simulink model "ExerciseModel_18072025"  (R2025a)
settings: Solver=ode4  StartTime=0.0  StopTime=tsim  FixedStep=1  RelTol=1e-3
model workspace (MAT data in the model file):
  step_size = 1
values from neighbouring files (symbols this model uses):
  A_w = [cosd(beta1)*sind(alfa1)  -cosd(beta2)*sind(alfa2) -cosd(beta3)*sind(alfa3) cosd(beta4)*sind(alfa4) ... (first row only)    [initfun_18072025.m]    (also in initfun_18072025_nogyro.m)
  A_wP = pinv(A_w)    [initfun_18072025.m]    (also in initfun_18072025_nogyro.m)
  ARW = deg2rad(0.23)/sqrt(3600)    [initfun_18072025.m]
  Bias = deg2rad(1)/3600    [initfun_18072025.m]
  C_d = 2.2    [initfun_18072025.m]    (also in initfun_18072025_nogyro.m)
  d_max = 0.29    [initfun_18072025.m]    (also in initfun_18072025_nogyro.m)
  d_min = 0    [initfun_18072025.m]    (also in initfun_18072025_nogyro.m)
  ET0 = cspice_str2et(Date_UTC)    [initfun_18072025.m]    (also in initfun_18072025_nogyro.m)
  FOV = 166    [initfun_18072025.m]    (also in initfun_18072025_nogyro.m)
  G_earth = 6.6742e-11    [initfun_18072025.m]    (also in initfun_18072025_nogyro.m)
  init_state = [initial_position,initial_velocity,ang_vel_init2,quat_0]'    [initfun_18072025.m]    (also in initfun_18072025_nogyro.m)
  K = [F Z(:); Z(:)' sigma]    [Gain_matrix.m]    (also in QUEST.m = Gain_matrix(V',W',a); initfun_18072025.m = schmidt(nmax, mmax); initfun_18072025_nogyro.m = schmidt(nmax, mmax))
  K_dp = K_d_pitch_1    [evaluate_gains.m]    (also in evaluate_gains_nogyro.m)
  K_dr = K_d_roll_1    [evaluate_gains.m]    (also in evaluate_gains_nogyro.m)
  K_dy = K_d_yaw_1    [evaluate_gains.m]    (also in evaluate_gains_nogyro.m)
  K_pp = K_p_pitch_1    [evaluate_gains.m]    (also in evaluate_gains_nogyro.m; initfun_18072025_nogyro.m = K_pp/2)
  K_pr = K_p_roll_1    [evaluate_gains.m]    (also in evaluate_gains_nogyro.m; initfun_18072025.m = K_pr*1.8)
  K_py = K_p_yaw_1    [evaluate_gains.m]    (also in evaluate_gains_nogyro.m; initfun_18072025.m = K_py*10)
  m_earth = 5.9736e24    (= 5.9736e+24)    [initfun_18072025.m]    (also in initfun_18072025_nogyro.m)
  Magnetic_dipole = [0.1; 0.1;  0.1]    [initfun_18072025.m]    (also in initfun_18072025_nogyro.m)
  Magnetometers_number = 2    [initfun_18072025.m]    (also in initfun_18072025_nogyro.m)
  Mean_cart_Mag = 0    [initfun_18072025.m]    (also in initfun_18072025_nogyro.m)
  MeanangularSun = 0    [initfun_18072025.m]    (also in initfun_18072025_nogyro.m)
  mmax = 3    [initfun_18072025.m]    (also in initfun_18072025_nogyro.m)
  nmax = 3    [initfun_18072025.m]    (also in initfun_18072025_nogyro.m)
  omegaOrb = [0;-2*pi/P;0]    [initfun_18072025.m]    (also in initfun_18072025_nogyro.m)
  P_prev = [P_dg, zeros(3,3) ... (first row only)    [initfun_18072025.m]    (also in initfun_18072025_nogyro.m)
  P_sun = 4.56e-6    (= 4.56e-06)    [initfun_18072025.m]    (also in initfun_18072025_nogyro.m)
  Q = [eye(3,3).*Qattitudefactor zeros(3,3) ... (first row only)    [initfun_18072025.m]    (also in initfun_18072025_nogyro.m)
  R_B = (Sigma_cart_Mag)^2    (= 2.77777777778e-16)    [initfun_18072025.m]    (also in initfun_18072025_nogyro.m)
  r_earth = 6371e3    (= 6371000)    [initfun_18072025.m]    (also in initfun_18072025_nogyro.m)
  R_G = ARW^2    [initfun_18072025.m]
  R_SS = (SigmaangularSun*pi/180)^2    (= 3.04617419787e-06)    [initfun_18072025.m]    (also in initfun_18072025_nogyro.m)
  RWs_Inertia = diag([9.0718e-06, 9.0718e-06, 9.0718e-06, 9.0718e-06])    [initfun_18072025.m]    (also in initfun_18072025_nogyro.m)
  RWs_Inertia_Inv = inv(RWs_Inertia)    [initfun_18072025.m]    (also in initfun_18072025_nogyro.m)
  Sat_Inertia = diag([6.295, 1.644, 5.462]*10^-1)    [initfun_18072025.m]    (also in initfun_18072025_nogyro.m)
  Sat_mass = 12.172    [initfun_18072025.m]    (also in initfun_18072025_nogyro.m)
  Sigma_cart_Mag = (50*10^-9)/3    (= 1.66666666667e-08)    [initfun_18072025.m]    (also in initfun_18072025_nogyro.m)
  SigmaangularSun = 0.1    [initfun_18072025.m]    (also in initfun_18072025_nogyro.m)
  Sun_sensors = zeros(3, SS_number)    [initfun_18072025.m]    (also in initfun_18072025_nogyro.m)
  threshold_omega = omega_max * 0.8    (= 837.7580408)    [initfun_18072025.m]    (also in initfun_18072025_nogyro.m)
  x_prev = x0    [initfun_18072025.m]    (also in initfun_18072025_nogyro.m)
undefined symbols (not defined in the file or in its folder): DiscIntNeverNeededParam, G, H, IAU, juliandate, quat_feed_reg, Sat_Aeromodel_det
libraries: matrix_library x9, vrlib x2, aerolibtransform2 x1
(part 1 of 3)
settings Model: Creator=LaMar  LastModifiedBy=pietr
settings OptimizationCC: ReuseModelBlockBuffer=off
settings RTWCC: GPUComputeCapability=3.5

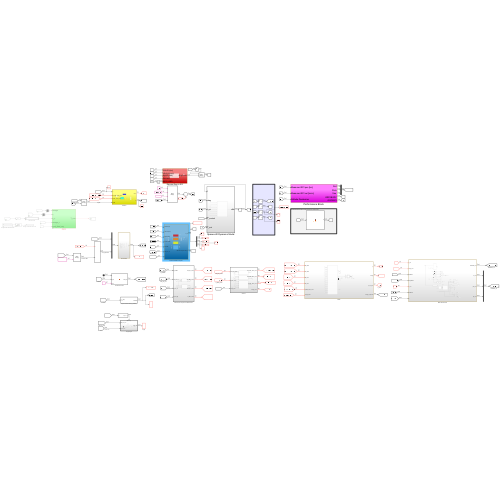
[thumbnail: Simulink's stored preview of the top-level diagram]
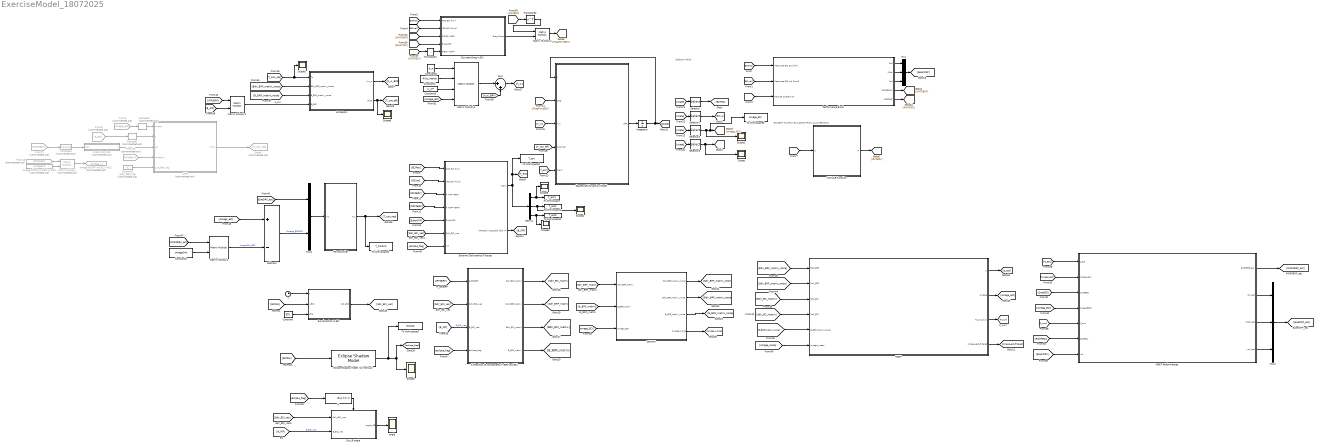
== system ExerciseModel_18072025 ==
  note: ECI2BRF MATRIX BUILDING FROM QUATERNION
  note: Selector Panel
  Actuators : Subsystem
  Constant : Constant  Value=ET0
  Constant2 : Constant  Commented=on  Value=quat_feed_reg  OutDataTypeStr=Bus: Quat_feed_reg
  Constant3 : Constant  Value=omegaOrb
  Constant4 : Constant  Value=RWs_Inertia
  Constant5 : Constant  Value=A_wP
  Constant6 : Constant  Value=A_w
  Demux : Demux  Outputs=3
  Discrete Drag in ECI : Subsystem
  Eclipse Shadow Model (Cylindrical) : EclipseShadowModel  units=Metric (km)  shadowModel=Cylindrical  startDate=juliandate(2025, 7, 23, 8, 30, 00)  includeMoon=off  ephemerisModel=DE430  useEphemerisDateRange=off
  External Disturbance Torques : Subsystem
  From17 : From  Commented=on  GotoTag=RORFECI
  From18 : From  Commented=on  GotoTag=RORFECI
  From19 : From  Commented=on  GotoTag=omega_c
  From5 : From  Commented=on  GotoTag=omega_est
  From6 : From  Commented=on  GotoTag=q_est
  Goto8 : Goto  Commented=on  GotoTag=T_con_req
  If : If  IfExpression=u1 == 1  ShowElse=off
  Integrator : Integrator  InitialCondition=init_state
  MATLAB Function : MATLAB Function  TreatAsAtomicUnit=on
  MEKF : Subsystem
  MEKF Performances : Subsystem
  Matrix Multiply : Product  Commented=on  Multiplication=Matrix(*)
  Matrix Multiply1 : Product  Multiplication=Matrix(*)
  Matrix Multiply2 : Product  Multiplication=Matrix(*)
  Matrix Multiply3 : Product  Inputs=4  Multiplication=Matrix(*)
  Matrix Multiply4 : Product  Multiplication=Matrix(*)
  Mux : Mux  Inputs=3
  Mux1 : Mux  Inputs=2
  Mux2 : Mux  Inputs=3
  PD controller : Subsystem
  "Performance Block " : Subsystem
  QFR : Subsystem  Commented=on
  Quat From Rot : MATLAB Function  Commented=on  TreatAsAtomicUnit=on
  Reshape : Reshape  Commented=on  OutputDimensionality=Column vector (2-D)
  Reshape1 : Reshape  Commented=on  OutputDimensionality=Column vector (2-D)
  "S direction, B components in BRF and ECI" : Subsystem
  Scope{,1..7} (8 alike) : Scope
      Scope settings: ActiveDisplayYMinimum=-1.0956085480018865  ActiveDisplayYMaximum=1.0958852189411159  DataLoggingVariableName=ScopeData6
      Scope1 settings: ActiveDisplayYMinimum=-0.0013938529149849089  ActiveDisplayYMaximum=0.00069381752156411482  DataLoggingVariableName=ScopeData7
      Scope2 settings: ActiveDisplayYMinimum=-0.12499999999999997  ActiveDisplayYMaximum=1.125  DataLoggingVariableName=ScopeData23
      Scope3 settings: ActiveDisplayYMinimum=-7.1614000633141769E-5  ActiveDisplayYMaximum=2.858496093881435E-5  DataLoggingVariableName=ScopeData27
      Scope4 settings: ActiveDisplayYMinimum=-1  ActiveDisplayYMaximum=1  DataLoggingVariableName=ScopeData29
      Scope5 settings: ActiveDisplayYMinimum=-2.2142475985885582E-7  ActiveDisplayYMaximum=5.1230127670874118E-7  DataLoggingVariableName=ScopeData30
      Scope6 settings: ActiveDisplayYMinimum=-1.0E+8  ActiveDisplayYMaximum=1  DataLoggingVariableName=ScopeData32
      Scope7 settings: ActiveDisplayYMinimum=-2.6634282014264469E-5  ActiveDisplayYMaximum=0.00020835981186267849  DataLoggingVariableName=ScopeData37
  Selector : Selector  InputPortWidth=13  IndexOptions=Index vector (dialog)  Indices=[1 2 3]  OutputSizes=1
  Selector1 : Selector  InputPortWidth=13  IndexOptions=Index vector (dialog)  Indices=[4 5 6]  OutputSizes=1
  Selector2 : Selector  InputPortWidth=13  IndexOptions=Index vector (dialog)  Indices=[7 8 9]  OutputSizes=1
  Selector3 : Selector  InputPortWidth=13  IndexOptions=Index vector (dialog)  Indices=[10 11 12 13]  OutputSizes=1
  Sensors : Subsystem
  Spacecraft Dynamics Model : Subsystem
  Subtract : Sum  Inputs=+-
  Sum : Sum  Inputs=|++
  Sun direction in ECI : MATLAB Function  TreatAsAtomicUnit=on
  Sun_B angle : Subsystem  TreatAsAtomicUnit=on
  To Workspace : ToWorkspace  VariableName=T_ext1  SaveFormat=Timeseries  SampleTime=-1
  To Workspace1 : ToWorkspace  VariableName=T_ext2  SaveFormat=Timeseries  SampleTime=-1
  To Workspace2 : ToWorkspace  VariableName=T_ext3  SaveFormat=Timeseries  SampleTime=-1
  To Workspace3 : ToWorkspace  VariableName=T_ext  SaveFormat=Timeseries  SampleTime=-1
  To Workspace4 : ToWorkspace  VariableName=T_Control  SaveFormat=Timeseries  SampleTime=-1
  To Workspace5 : ToWorkspace  VariableName=eclipse  SaveFormat=Timeseries  SampleTime=-1
  To Workspace6 : ToWorkspace  VariableName=omega_ECI  SaveFormat=Timeseries  SampleTime=-1
  Transpose : matrix_library/Transpose  Commented=on
  Transpose1 : matrix_library/Transpose
  Transpose2 : Math  Operator=transpose
  angle : Scope
      settings: ActiveDisplayYMinimum=-9.7641140829559632  ActiveDisplayYMaximum=194.35927047346718  DataLoggingVariableName=ScopeData39
  omega of ORF wrt ECI in ECI : Goto  Commented=on  GotoTag=omega_c
  omega of ORF wrt ECI in ORF : Constant  Commented=on  Value=omegaOrb
  t : Clock
  wires:
  Spacecraft Dynamics Model/1(dfdt) -> Integrator/1
  Integrator/1 -> Spacecraft Dynamics Model/1(f), [state]
  Selector/1 -> [ECIPos]
  Selector1/1 -> [ECIvel]
  [ECIPos] -> "Performance Block "/1(Measured ECI pos [km])
  [ECIvel] -> "Performance Block "/2(Measured ECI vel [km/s])
  [QuatECI] -> "Performance Block "/3("Attitude Quaternion ")
  [ECIPos] -> Discrete Drag in ECI/1(POS ECI [km])
  [ECIvel] -> Discrete Drag in ECI/2(VEL ECI [km/s])
  "Performance Block "/1(Roll) -> Mux/1
  "Performance Block "/2(Pitch) -> Mux/2
  "Performance Block "/3("Yaw ") -> Mux/3
  Selector3/1 -> Scope/1, [QuatECI]
  Selector2/1 -> Scope1/1, To Workspace6/1, [omega_ECI]
  From5/1 -> Reshape1/1
  From6/1 -> Reshape/1
  Constant2/1 -> QFR/5(quat_feed_reg)
  [ECIPos] -> External Disturbance Torques/1(POS ECI [km])
  [ECIvel] -> External Disturbance Torques/2(VEL ECI [km/s])
  [IRF2BRF] -> External Disturbance Torques/3("R (IRF->BRF) ")
  [ORF2BRF] -> External Disturbance Torques/4("R (ORF->BRF) ")
  "Performance Block "/4(ORF2BODY) -> [ORF2BRF]
  MATLAB Function/1(R) -> [IRF2BRF]
  [QuatECI] -> MATLAB Function/1(q)
  Discrete Drag in ECI/1(Drag Force) -> Matrix Multiply4/2
  [T_ext] -> Spacecraft Dynamics Model/5(T_ext)
  [DragForceECI] -> Spacecraft Dynamics Model/2(drag)
  [h_w] -> Spacecraft Dynamics Model/3(h_w)
  [T_con_req] -> Scope7/1, Actuators/1(Tc)
  "Performance Block "/5(ORF2ECI) -> [RORFECI]
  Quat From Rot/1(q) -> QFR/3(q_c)
  From17/1 -> Transpose/1
  Transpose/1 -> Quat From Rot/1(dcm)
  From18/1 -> Matrix Multiply/1
  omega of ORF wrt ECI in ORF/1 -> Matrix Multiply/2
  Matrix Multiply/1 -> omega of ORF wrt ECI in ECI/1
  From19/1 -> QFR/4(omega_c)
  [ORF2BRF] -> Discrete Drag in ECI/3(R(ORF->BRF))
  [state] -> Selector/1
  [state] -> Selector3/1
  [state] -> Selector2/1
  [state] -> Selector1/1
  Mux/1 -> [EulerORF]
  [EulerORF] -> Discrete Drag in ECI/4(EulerORF)
  [RORFECI] -> Transpose1/1
  Transpose1/1 -> Discrete Drag in ECI/5(R(ECI->ORF))
  External Disturbance Torques/2(IRF Earth magnetic field (T)) -> [B_IRF]
  "S direction, B components in BRF and ECI"/3(Bdir_ECI_matrix) -> [Bdir_ECI_matrix]
  "S direction, B components in BRF and ECI"/1(Sdir_ECI_matrix) -> [Sdir_ECI_matrix]
  "S direction, B components in BRF and ECI"/2(Sdir_BRF_matrix) -> [Sdir_BRF_matrix]
  "S direction, B components in BRF and ECI"/4(B_BRF_matrix) -> [B_BRF_matrix]
  [Sdir_BRF_matrix] -> Sensors/1(Sdir_BRF_matrix)
  [B_BRF_matrix] -> Sensors/2(B_BRF_matrix)
  Sensors/2(Bdir_BRF_matrix_noise) -> [Bdir_BRF_matrix_noise]
  Sensors/1(Sdir_BRF_matrix_noise) -> [Sdir_BRF_matrix_noise]
  [B_IRF] -> "S direction, B components in BRF and ECI"/3(B_ECI_vec)  "B_ECI_vec"
  Constant/1 -> Sun direction in ECI/3(ET0)
  t/1 -> Sun direction in ECI/1(t)
  Sun direction in ECI/1(Sdir_ECI) -> [Sdir_ECI_vec]
  [ECIPos] -> Sun direction in ECI/2(r_ECI)
  [Bdir_ECI_matrix] -> MEKF/3(Bdir_ECI)
  MEKF/1(q) -> [q_est]
  MEKF/2(omega) -> [omega_est]
  [Bdir_BRF_matrix_noise] -> MEKF/1(Bdir_BRF)
  [Sdir_BRF_matrix_noise] -> MEKF/2(Sdir_BRF)
  [Sdir_ECI_matrix] -> MEKF/4(Sdir_ECI)
  [q_est] -> MEKF Performances/1(q_est)
  [omega_est] -> MEKF Performances/2(omega_est)
  [QuatECI] -> MEKF Performances/3(quatBECI)
  [omega_ECI] -> MEKF Performances/4(omegaBECI)
  MEKF/3(P_curr_plus) -> [P_curr]
  [P_curr] -> MEKF Performances/5(P_curr)
  [EulerORF] -> MEKF Performances/7(In8)
  [RORFECI] -> MEKF Performances/6(RORFECI)
  [Bdir_BRF_matrix_noise] -> Actuators/2(Bdir_BRF_matrix_noise)
  Sensors/3(B_BRF_matrix_noise) -> [B_BRF_matrix_noise]
  [B_BRF_matrix_noise] -> MEKF/5(B_BRF_matrix_noise)
  [B_BRF_matrix_noise] -> Actuators/3(B_BRF_matrix_noise)
  [B_IRF] -> Matrix Multiply1/2
  [IRF2BRF] -> Matrix Multiply1/1
  Matrix Multiply1/1 -> Actuators/4(B_BRF)  "B_BRF"
  Actuators/2(Out1) -> Scope6/1, [T_con_eff]
  [ECIPos] -> Eclipse Shadow Model (Cylindrical)/1
  Constant3/1 -> Matrix Multiply2/2
  [RORFBRF_est] -> Matrix Multiply2/1
  Matrix Multiply2/1 -> Subtract/2  "omegaOrb_BRF"
  Subtract/1 -> Mux1/2  "Omega_BRFORF"
  [EuleORF_est] -> Mux1/1
  Mux1/1 -> PD controller/1(In1)
  PD controller/1(T_c) -> To Workspace4/1, [T_con_req]
  [IRF2BRF] -> "S direction, B components in BRF and ECI"/1(R_ECIBRF)
  [Sdir_ECI_vec] -> "S direction, B components in BRF and ECI"/2(Sdir_ECI_vec)
  [Sdir_ECI_vec] -> External Disturbance Torques/6(Sdir_ECI_vec)
  [eclipse_flag] -> "S direction, B components in BRF and ECI"/4(eclipse_flag)
  [eclipse_flag] -> External Disturbance Torques/7(In7)
  External Disturbance Torques/1(T_ext) -> To Workspace3/1, [T_ext], Demux/1
  Demux/1 -> Scope5/1, To Workspace/1
  Demux/2 -> Scope4/1, To Workspace1/1
  Demux/3 -> Scope3/1, To Workspace2/1
  [T_con_eff] -> Spacecraft Dynamics Model/4(T_control)
  [EulerORF] -> External Disturbance Torques/5(EulerORF)
  [omega_ECI] -> Matrix Multiply3/4
  Constant5/1 -> Matrix Multiply3/3
  Matrix Multiply3/1 -> Sum/1
  Constant4/1 -> Matrix Multiply3/2
  Sum/1 -> [h_w]
  Constant6/1 -> Matrix Multiply3/1
  Actuators/1(hw_w) -> [h_w_BRF]
  [h_w_BRF] -> Sum/2
  QFR/1(T_con) -> Goto8/1
  Sun_B angle/1(angle_SB) -> angle/1
  If/1 -> Sun_B angle/Action
  [eclipse_flag] -> If/1
  [Sdir_ECI_vec] -> Sun_B angle/1(Sdir_ECI_vec)
  [B_IRF] -> Sun_B angle/2(B_ECI_vec)  "B_ECI_vec"
  MEKF Performances/4(yaw_est) -> Mux2/3
  MEKF Performances/3(pitch_est) -> Mux2/2
  MEKF Performances/2(roll_est) -> Mux2/1
  MEKF Performances/1(RORFBRF_est) -> [RORFBRF_est]
  Mux2/1 -> [EuleORF_est]
  [omega_est] -> Subtract/1
  MEKF/4(omega_est_filtered) -> [omega_est_filtered]
  Reshape/1 -> QFR/2(q)
  Reshape1/1 -> QFR/1(omega)
  [omega_ECI] -> Sensors/3(omega_ECI)
  Sensors/4(omega_noise) -> [omega_noise]
  [omega_noise] -> MEKF/6(omega_meas)
  Eclipse Shadow Model (Cylindrical)/1 -> To Workspace5/1, Scope2/1, [eclipse_flag]
  [IRF2BRF] -> Transpose2/1
  Transpose2/1 -> Matrix Multiply4/1
  Matrix Multiply4/1 -> [DragForceECI]

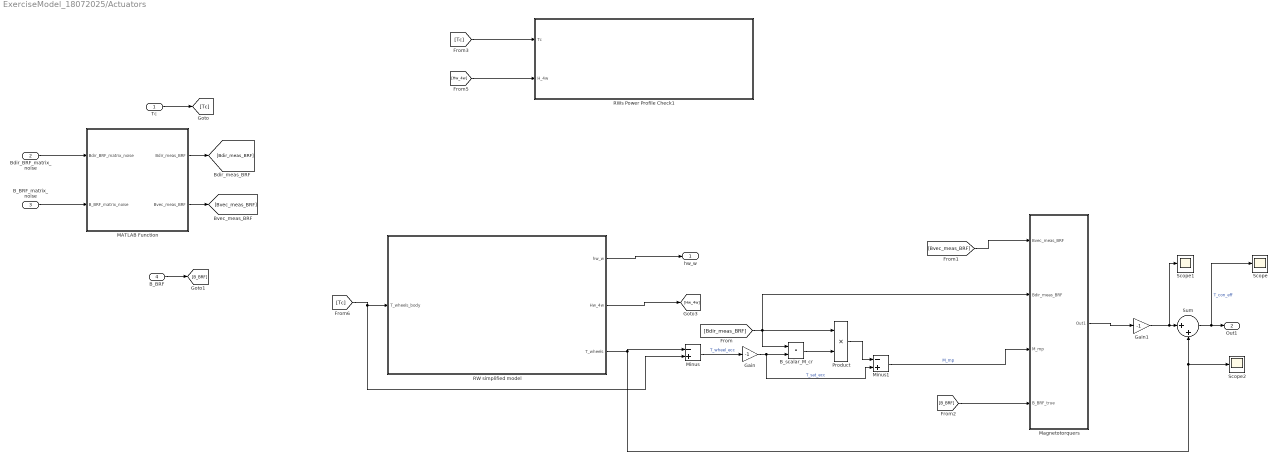
== system ExerciseModel_18072025/Actuators ==
  Tc : Inport
  Bdir_BRF_matrix_noise : Inport  Port=2
  B_BRF_matrix_noise : Inport  Port=3
  B_BRF : Inport  Port=4
  B_scalar_M_cr : DotProduct  OutDataTypeStr=Inherit: Inherit via internal rule
  Gain : Gain  Gain=-1
  Gain1 : Gain  Gain=-1
  MATLAB Function : MATLAB Function  TreatAsAtomicUnit=on
  Magnetotorquers : Subsystem
  Minus : Sum  Inputs=-+
  Minus1 : Sum  Inputs=-+
  Product : Product
  RW simplified model : Subsystem
  RWs Power Profile Check1 : Subsystem
  Scope : Scope
      settings: ActiveDisplayYMinimum=-1.8787661900659558E-5  ActiveDisplayYMaximum=1.7178053989984975E-5  DataLoggingVariableName=ScopeData33
  Scope1 : Scope
      settings: ActiveDisplayYMinimum=-8.6936992536621968E-6  ActiveDisplayYMaximum=1.5293515542539849E-5  DataLoggingVariableName=ScopeData34
  Scope2 : Scope
      settings: ActiveDisplayYMinimum=0.78642649193316594  ActiveDisplayYMaximum=0.98839878694816619  DataLoggingVariableName=ScopeData35
  Sum : Sum  Inputs=|++
  hw_w : Outport
  Out1 : Outport  Port=2
  wires:
  RW simplified model/3(T_wheels) -> Minus/1, Scope2/1, Sum/2
  Minus/1 -> Gain/1  "T_wheel_ecc"
  Gain/1 -> Minus1/2, B_scalar_M_cr/2  "T_sat_ecc"
  RW simplified model/1(hw_w) -> hw_w/1
  [Tc] -> Minus/2, RW simplified model/1(T_wheels_body)
  [Tc] -> RWs Power Profile Check1/1(Tc)
  RW simplified model/2(Hw_4w) -> [Hw_4w]
  [Hw_4w] -> RWs Power Profile Check1/2(H_4w)
  Tc/1 -> [Tc]
  Bdir_BRF_matrix_noise/1 -> MATLAB Function/1(Bdir_BRF_matrix_noise)
  MATLAB Function/1(Bdir_meas_BRF) -> [Bdir_meas_BRF]
  [Bdir_meas_BRF] -> B_scalar_M_cr/1, Magnetotorquers/2(Bdir_meas_BRF), Product/1
  B_scalar_M_cr/1 -> Product/2
  Product/1 -> Minus1/1
  Minus1/1 -> Magnetotorquers/3(M_mp)  "M_mp"
  B_BRF_matrix_noise/1 -> MATLAB Function/2(B_BRF_matrix_noise)
  MATLAB Function/2(Bvec_meas_BRF) -> [Bvec_meas_BRF]
  [Bvec_meas_BRF] -> Magnetotorquers/1(Bvec_meas_BRF)
  B_BRF/1 -> [B_BRF]
  [B_BRF] -> Magnetotorquers/4(B_BRF_true)
  Magnetotorquers/1(Out1) -> Gain1/1
  Gain1/1 -> Scope1/1, Sum/1
  Sum/1 -> Scope/1, Out1/1  "T_con_eff"

== system ExerciseModel_18072025/Discrete Drag in ECI ==
  POS ECI [km] : Inport
  VEL ECI [km/s] : Inport  Port=2
  R(ORF->BRF) : Inport  Port=3
  EulerORF : Inport  Port=4
  R(ECI->ORF) : Inport  Port=5
  DRAG FORCE IN ORF [N] : Subsystem
  Display : Display
  Matrix Multiply : Product  Multiplication=Matrix(*)
  Drag Force : Outport
  wires:
  R(ORF->BRF)/1 -> [RORFBRF]
  VEL ECI [km/s]/1 -> DRAG FORCE IN ORF [N]/2(Velocity  (V))
  POS ECI [km]/1 -> DRAG FORCE IN ORF [N]/1(Position (X))
  DRAG FORCE IN ORF [N]/1(Drag) -> Matrix Multiply/2
  Matrix Multiply/1 -> Display/1, Drag Force/1
  [RORFBRF] -> Matrix Multiply/1
  EulerORF/1 -> DRAG FORCE IN ORF [N]/3(EulerORF)
  [RECI2ORF] -> DRAG FORCE IN ORF [N]/4(ECI2ORF)
  R(ECI->ORF)/1 -> [RECI2ORF]

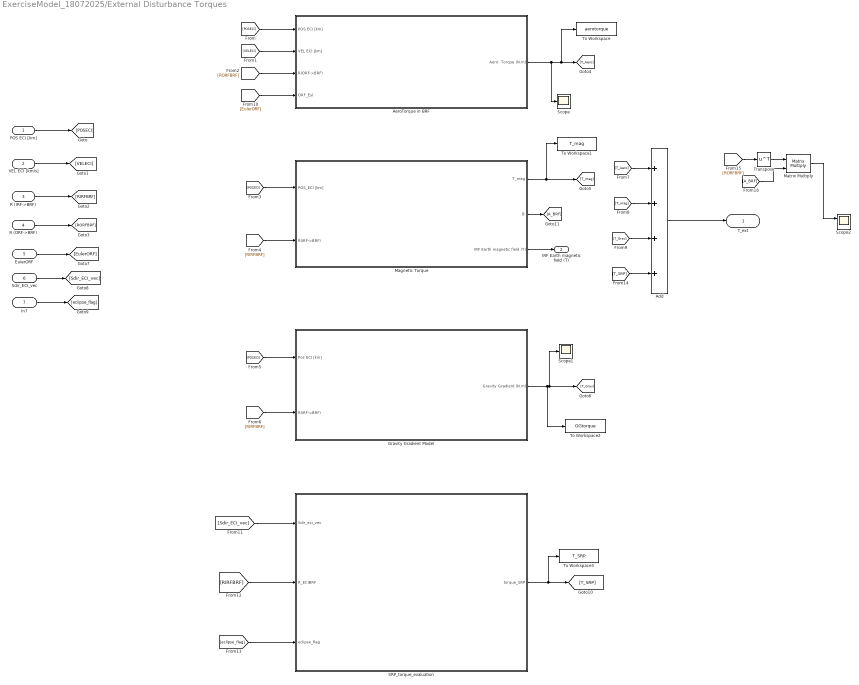
== system ExerciseModel_18072025/External Disturbance Torques ==
  POS ECI [km] : Inport
  VEL ECI [km/s] : Inport  Port=2
  "R (IRF->BRF) " : Inport  Port=3
  "R (ORF->BRF) " : Inport  Port=4
  EulerORF : Inport  Port=5
  Sdir_ECI_vec : Inport  Port=6
  In7 : Inport  Port=7
  Add : Sum  Inputs=++++
  AeroTorque in BRF : Subsystem
  Gravity Gradient Model : Subsystem
  Magnetic Torque : Subsystem
  Matrix Multiply : Product  Multiplication=Matrix(*)
  SRP_torque_evaluation : Subsystem
  Scope : Scope
      settings: ActiveDisplayYMinimum=-0.0073443366381598105  ActiveDisplayYMaximum=0.0061896582898468347  DataLoggingVariableName=ScopeData28
  Scope1 : Scope
      settings: ActiveDisplayYMinimum=-7.59224298580784E-9  ActiveDisplayYMaximum=6.836938535445761E-9  DataLoggingVariableName=ScopeData31
  Scope2 : Scope  NumInputPorts=2
      settings: ActiveDisplayYMinimum=-5.8615088581894655E-5  ActiveDisplayYMaximum=5.8159689597254534E-5  DataLoggingVariableName=ScopeData42
  To Workspace : ToWorkspace  VariableName=aerotorque  SaveFormat=Timeseries  SampleTime=-1
  To Workspace1 : ToWorkspace  VariableName=T_mag  SaveFormat=Timeseries  SampleTime=-1
  To Workspace2 : ToWorkspace  VariableName=GGtorque  SaveFormat=Timeseries  SampleTime=-1
  To Workspace3 : ToWorkspace  VariableName=T_SRP  SaveFormat=Timeseries  SampleTime=-1
  Transpose : Math  Operator=transpose
  T_ext : Outport
  IRF Earth magnetic field (T) : Outport  Port=2
  wires:
  POS ECI [km]/1 -> [POSECI]
  VEL ECI [km/s]/1 -> [VELECI]
  "R (IRF->BRF) "/1 -> [RIRFBRF]
  "R (ORF->BRF) "/1 -> [RORFBRF]
  [POSECI] -> AeroTorque in BRF/1(POS ECI [km])
  [VELECI] -> AeroTorque in BRF/2(VEL ECI [km])
  [RORFBRF] -> AeroTorque in BRF/3(R(ORF->BRF))
  [POSECI] -> Magnetic Torque/1(POS_ECI [km])
  [RIRFBRF] -> Magnetic Torque/2(R(IRF->BRF))
  [RIRFBRF] -> Gravity Gradient Model/2(R(IRF->BRF))
  [POSECI] -> Gravity Gradient Model/1(Pos ECI [km])
  AeroTorque in BRF/1(Aero. Torque (N.m)) -> Scope/1, To Workspace/1, [T_Aero]
  Magnetic Torque/1(T_mag) -> To Workspace1/1, [T_mag]
  Magnetic Torque/2(B) -> [A_BRF]
  Gravity Gradient Model/1(Gravity Gradient (N.m)) -> To Workspace2/1, Scope1/1, [T_Grav]
  Add/1 -> T_ext/1
  [T_Aero] -> Add/1
  [T_Grav] -> Add/3
  [T_mag] -> Add/2
  [EulerORF] -> AeroTorque in BRF/4(ORF_Eul)
  EulerORF/1 -> [EulerORF]
  Sdir_ECI_vec/1 -> [Sdir_ECI_vec]
  [Sdir_ECI_vec] -> SRP_torque_evaluation/1(Sdir_eci_vec)
  [RIRFBRF] -> SRP_torque_evaluation/2(R_ECIBRF)
  In7/1 -> [eclipse_flag]
  [eclipse_flag] -> SRP_torque_evaluation/3(eclipse_flag)
  SRP_torque_evaluation/1(torque_SRP) -> To Workspace3/1, [T_SRP]
  [T_SRP] -> Add/4
  Magnetic Torque/3(IRF Earth magnetic field (T)) -> IRF Earth magnetic field (T)/1
  [RORFBRF] -> Transpose/1
  Transpose/1 -> Matrix Multiply/1
  [A_BRF] -> Matrix Multiply/2
  Matrix Multiply/1 -> Scope2/1

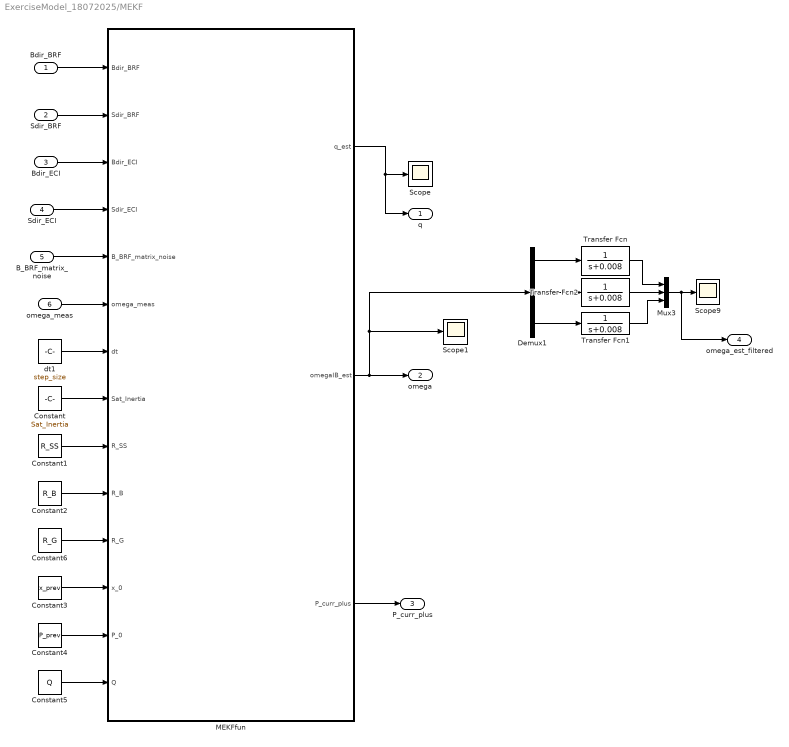
== system ExerciseModel_18072025/MEKF ==
  Bdir_BRF : Inport
  Sdir_BRF : Inport  Port=2
  Bdir_ECI : Inport  Port=3
  Sdir_ECI : Inport  Port=4
  B_BRF_matrix_noise : Inport  Port=5
  omega_meas : Inport  Port=6
  Constant : Constant  Value=Sat_Inertia
  Constant1 : Constant  Value=R_SS
  Constant2 : Constant  Value=R_B
  Constant3 : Constant  Value=x_prev
  Constant4 : Constant  Value=P_prev
  Constant5 : Constant  Value=Q
  Constant6 : Constant  Value=R_G
  Demux1 : Demux  Outputs=3
  MEKFfun : MATLAB Function  TreatAsAtomicUnit=on
  Mux3 : Mux  Inputs=3
  Scope : Scope
      settings: ActiveDisplayYMinimum=0.069030538530036489  ActiveDisplayYMaximum=0.56351563715965813  DataLoggingVariableName=ScopeData4
  Scope1 : Scope
      settings: ActiveDisplayYMinimum=-0.0014038743390512374  ActiveDisplayYMaximum=0.00035853988806748744  DataLoggingVariableName=ScopeData5
  Scope9 : Scope
      settings: ActiveDisplayYMinimum=-0.35053277395134796  ActiveDisplayYMaximum=0.58026887260329929  DataLoggingVariableName=ScopeData40
  Transfer Fcn : TransferFcn  Denominator=[1 0.008]
  Transfer Fcn1 : TransferFcn  Denominator=[1 0.008]
  Transfer Fcn2 : TransferFcn  Denominator=[1 0.008]
  dt1 : Constant  Value=step_size
  q : Outport
  omega : Outport  Port=2
  P_curr_plus : Outport  Port=3
  omega_est_filtered : Outport  Port=4
  wires:
  MEKFfun/1(q_est) -> q/1, Scope/1
  Constant3/1 -> MEKFfun/12(x_0)
  dt1/1 -> MEKFfun/7(dt)
  Bdir_BRF/1 -> MEKFfun/1(Bdir_BRF)
  Constant5/1 -> MEKFfun/14(Q)
  Constant4/1 -> MEKFfun/13(P_0)
  Bdir_ECI/1 -> MEKFfun/3(Bdir_ECI)
  Sdir_ECI/1 -> MEKFfun/4(Sdir_ECI)
  Sdir_BRF/1 -> MEKFfun/2(Sdir_BRF)
  Constant/1 -> MEKFfun/8(Sat_Inertia)
  Constant2/1 -> MEKFfun/10(R_B)
  Constant1/1 -> MEKFfun/9(R_SS)
  MEKFfun/3(P_curr_plus) -> P_curr_plus/1
  B_BRF_matrix_noise/1 -> MEKFfun/5(B_BRF_matrix_noise)
  Demux1/1 -> Transfer Fcn/1
  Transfer Fcn2/1 -> Mux3/2
  Transfer Fcn/1 -> Mux3/1
  Transfer Fcn1/1 -> Mux3/3
  Demux1/3 -> Transfer Fcn1/1
  Mux3/1 -> omega_est_filtered/1, Scope9/1
  MEKFfun/2(omegaIB_est) -> Demux1/1, Scope1/1, omega/1
  Demux1/2 -> Transfer Fcn2/1
  Constant6/1 -> MEKFfun/11(R_G)
  omega_meas/1 -> MEKFfun/6(omega_meas)

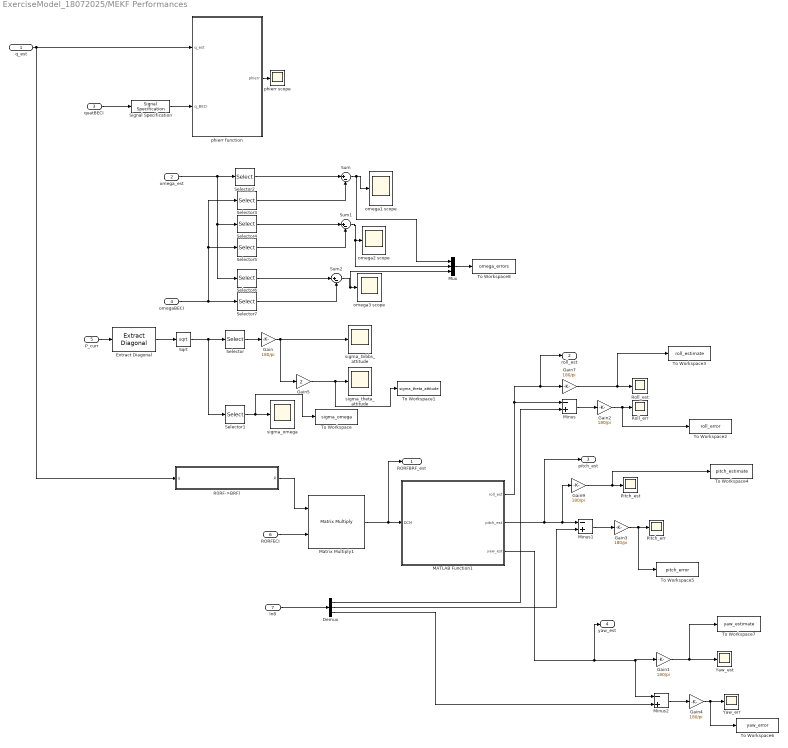
== system ExerciseModel_18072025/MEKF Performances ==
  q_est : Inport
  omega_est : Inport  Port=2
  quatBECI : Inport  Port=3
  omegaBECI : Inport  Port=4
  P_curr : Inport  Port=5
  RORFECI : Inport  Port=6
  In8 : Inport  Port=7
  Demux : Demux  Outputs=3
  Extract Diagonal : matrix_library/Extract Diagonal
      settings: LibrarySourceBlock=|
      | simulink/Matrix
      | Operations/Extract Diagonal
  Gain{,1..4,7,9} (7 alike) : Gain  Gain=180/pi
  Gain5 : Gain  Gain=2
  MATLAB Function1 : MATLAB Function  TreatAsAtomicUnit=on
  Matrix Multiply1 : Product  Multiplication=Matrix(*)
  Minus : Sum  Inputs=-+
  Minus1 : Sum  Inputs=-+
  Minus2 : Sum  Inputs=-+
  Mux : Mux  Inputs=3
  Pitch_err : Scope
      settings: ActiveDisplayYMinimum=-0.04628003954738745  ActiveDisplayYMaximum=0.034432404258830158  DataLoggingVariableName=ScopeData9
  Pitch_est : Scope
      settings: ActiveDisplayYMinimum=-90.1418838729579  ActiveDisplayYMaximum=-74.2068735641986  DataLoggingVariableName=ScopeData17
  R(IRF->BRF) : MATLAB Function  TreatAsAtomicUnit=on
  Roll_err : Scope
      settings: ActiveDisplayYMinimum=-0.085460707156846713  ActiveDisplayYMaximum=0.033420462421589622  DataLoggingVariableName=ScopeData8
  Roll_est : Scope
      settings: ActiveDisplayYMinimum=-0.22501522229156135  ActiveDisplayYMaximum=0.32261161883110218  DataLoggingVariableName=ScopeData19
  Selector : Selector  InputPortWidth=6  IndexOptions=Index vector (dialog)  Indices=[1 2 3]  OutputSizes=1
  Selector1 : Selector  InputPortWidth=6  IndexOptions=Index vector (dialog)  Indices=[4 5 6]  OutputSizes=1
  Selector2 : Selector  InputPortWidth=3  IndexOptions=Index vector (dialog)  Indices=[1]  OutputSizes=1
  Selector3 : Selector  InputPortWidth=3  IndexOptions=Index vector (dialog)  Indices=[1]  OutputSizes=1
  Selector4 : Selector  InputPortWidth=3  IndexOptions=Index vector (dialog)  Indices=[2]  OutputSizes=1
  Selector5 : Selector  InputPortWidth=3  IndexOptions=Index vector (dialog)  Indices=[2]  OutputSizes=1
  Selector6 : Selector  InputPortWidth=3  IndexOptions=Index vector (dialog)  Indices=[3]  OutputSizes=1
  Selector7 : Selector  InputPortWidth=3  IndexOptions=Index vector (dialog)  Indices=[3]  OutputSizes=1
  Signal Specification : SignalSpecification  Dimensions=[1,4]  SampleTime=step_size
  Sqrt : Sqrt
  Sum : Sum  Inputs=|+-
  Sum1 : Sum  Inputs=|+-
  Sum2 : Sum  Inputs=|+-
  To Workspace : ToWorkspace  VariableName=sigma_omega  SaveFormat=Timeseries  SampleTime=-1
  To Workspace1 : ToWorkspace  VariableName=sigma_theta_attitude  SaveFormat=Timeseries  SampleTime=-1
  To Workspace2 : ToWorkspace  VariableName=roll_error  SaveFormat=Timeseries  SampleTime=-1
  To Workspace3 : ToWorkspace  VariableName=roll_estimate  SaveFormat=Timeseries  SampleTime=-1
  To Workspace4 : ToWorkspace  VariableName=pitch_estimate  SaveFormat=Timeseries  SampleTime=-1
  To Workspace5 : ToWorkspace  VariableName=pitch_error  SaveFormat=Timeseries  SampleTime=-1
  To Workspace6 : ToWorkspace  VariableName=yaw_error  SaveFormat=Timeseries  SampleTime=-1
  To Workspace7 : ToWorkspace  VariableName=yaw_estimate  SaveFormat=Timeseries  SampleTime=-1
  To Workspace8 : ToWorkspace  VariableName=omega_errors  SaveFormat=Timeseries  SampleTime=-1
  Yaw_err : Scope
      settings: ActiveDisplayYMinimum=-0.0350952720791284  ActiveDisplayYMaximum=0.040618860650201559  DataLoggingVariableName=ScopeData10
  Yaw_est : Scope
      settings: ActiveDisplayYMinimum=-1.4595386804960515  ActiveDisplayYMaximum=3.0244410200738057  DataLoggingVariableName=ScopeData18
  omega1 scope : Scope
      settings: ActiveDisplayYMinimum=-0.00029654727329008238  ActiveDisplayYMaximum=0.0003358495705412497  DataLoggingVariableName=ScopeData12
  omega2 scope : Scope
      settings: ActiveDisplayYMinimum=-0.00033833740814389685  ActiveDisplayYMaximum=0.00035071490718946132  DataLoggingVariableName=ScopeData15
  omega3 scope : Scope
      settings: ActiveDisplayYMinimum=-0.00037236545009210989  ActiveDisplayYMaximum=0.0004491218895278383  DataLoggingVariableName=ScopeData16
  phierr function : MATLAB Function  TreatAsAtomicUnit=on
  phierr scope : Scope
      settings: ActiveDisplayYMinimum=-19.85603860338669  ActiveDisplayYMaximum=178.71348738740437  DataLoggingVariableName=ScopeData11
  sigma_Gibbs_attitude : Scope
      settings: ActiveDisplayYMinimum=-0.0030338730248680003  ActiveDisplayYMaximum=0.058243365546428068  DataLoggingVariableName=ScopeData13
  sigma_omega : Scope
      settings: ActiveDisplayYMinimum=6.5429909136817193E-5  ActiveDisplayYMaximum=6.6231154434048621E-5  DataLoggingVariableName=ScopeData14
  sigma_theta_attitude : Scope
      settings: ActiveDisplayYMinimum=-0.0024031340685375137  ActiveDisplayYMaximum=0.092216390918461233  DataLoggingVariableName=ScopeData38
  RORFBRF_est : Outport
  roll_est : Outport  Port=2
  pitch_est : Outport  Port=3
  yaw_est : Outport  Port=4
  wires:
  quatBECI/1 -> Signal Specification/1
  Signal Specification/1 -> phierr function/2(q_BECI)
  phierr function/1(phierr) -> phierr scope/1
  P_curr/1 -> Extract Diagonal/1
  Extract Diagonal/1 -> Sqrt/1
  Sqrt/1 -> Selector/1, Selector1/1
  Selector1/1 -> To Workspace/1, sigma_omega/1
  omega_est/1 -> Selector6/1, Selector4/1, Selector2/1
  omegaBECI/1 -> Selector7/1, Selector5/1, Selector3/1
  Selector2/1 -> Sum/1
  Selector3/1 -> Sum/2
  Selector4/1 -> Sum1/1
  Selector5/1 -> Sum1/2
  Selector6/1 -> Sum2/1
  Selector7/1 -> Sum2/2
  R(IRF->BRF)/1(R) -> Matrix Multiply1/1
  MATLAB Function1/1(roll_est) -> roll_est/1, Gain7/1, Minus/1
  MATLAB Function1/2(pitch_est) -> pitch_est/1, Minus1/1, Gain9/1
  q_est/1 -> R(IRF->BRF)/1(q), phierr function/1(q_est)
  MATLAB Function1/3(yaw_est) -> yaw_est/1, Minus2/1, Gain1/1
  Matrix Multiply1/1 -> RORFBRF_est/1, MATLAB Function1/1(DCM)
  Gain7/1 -> To Workspace3/1, Roll_est/1
  Gain1/1 -> To Workspace7/1, Yaw_est/1
  RORFECI/1 -> Matrix Multiply1/2
  Gain9/1 -> To Workspace4/1, Pitch_est/1
  In8/1 -> Demux/1
  Demux/1 -> Minus/2
  Minus/1 -> Gain2/1
  Gain2/1 -> To Workspace2/1, Roll_err/1
  Minus1/1 -> Gain3/1
  Gain3/1 -> To Workspace5/1, Pitch_err/1
  Demux/2 -> Minus1/2
  Minus2/1 -> Gain4/1
  Gain4/1 -> To Workspace6/1, Yaw_err/1
  Demux/3 -> Minus2/2
  Selector/1 -> Gain/1
  Gain/1 -> Gain5/1, sigma_Gibbs_attitude/1
  Gain5/1 -> To Workspace1/1, sigma_theta_attitude/1
  Sum/1 -> Mux/1, omega1 scope/1
  Sum1/1 -> omega2 scope/1, Mux/2
  Sum2/1 -> Mux/3, omega3 scope/1
  Mux/1 -> To Workspace8/1

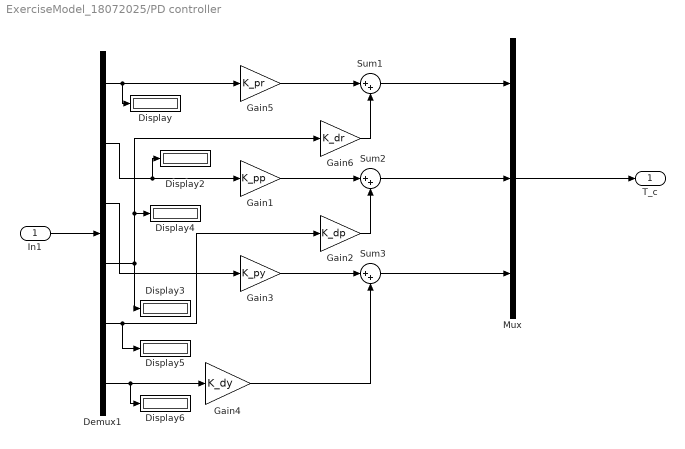
== system ExerciseModel_18072025/PD controller ==
  In1 : Inport
  Demux1 : Demux  Outputs=6
  Display{,2..6} (6 alike) : Display
  Gain1 : Gain  Gain=K_pp
  Gain2 : Gain  Gain=K_dp
  Gain3 : Gain  Gain=K_py
  Gain4 : Gain  Gain=K_dy
  Gain5 : Gain  Gain=K_pr
  Gain6 : Gain  Gain=K_dr
  Mux : Mux  Inputs=3
  Sum1 : Sum  Inputs=|++
  Sum2 : Sum  Inputs=|++
  Sum3 : Sum  Inputs=|++
  T_c : Outport
  wires:
  Gain2/1 -> Sum2/2
  Demux1/1 -> Display/1, Gain5/1
  Gain1/1 -> Sum2/1
  Gain4/1 -> Sum3/2
  Sum2/1 -> Mux/2
  Demux1/6 -> Display6/1, Gain4/1
  Demux1/2 -> Display2/1, Gain1/1
  Demux1/3 -> Gain3/1
  In1/1 -> Demux1/1
  Sum1/1 -> Mux/1
  Gain5/1 -> Sum1/1
  Sum3/1 -> Mux/3
  Demux1/4 -> Display4/1, Gain6/1, Display3/1
  Gain3/1 -> Sum3/1
  Gain6/1 -> Sum1/2
  Mux/1 -> T_c/1
  Demux1/5 -> Gain2/1, Display5/1

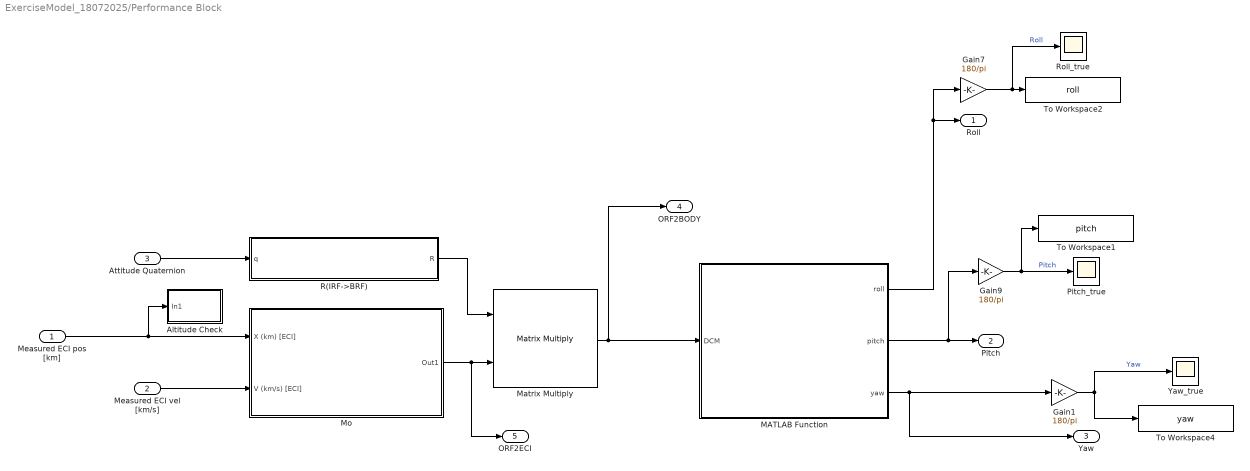
== system ExerciseModel_18072025/Performance Block  ==
  Measured ECI pos [km] : Inport
  Measured ECI vel [km/s] : Inport  Port=2
  "Attitude Quaternion " : Inport  Port=3
  Altitude Check : Subsystem
  Gain1 : Gain  Gain=180/pi
  Gain7 : Gain  Gain=180/pi
  Gain9 : Gain  Gain=180/pi
  MATLAB Function : MATLAB Function  TreatAsAtomicUnit=on
  Matrix Multiply : Product  Multiplication=Matrix(*)
  Mo : Subsystem
  Pitch_true : Scope
      settings: TimeSpan=100  ActiveDisplayYMinimum=-0.35626182860394795  ActiveDisplayYMaximum=0.25218220221437149
  R(IRF->BRF) : MATLAB Function  TreatAsAtomicUnit=on
  Roll_true : Scope
      settings: ActiveDisplayYMinimum=-0.33745974250061544  ActiveDisplayYMaximum=0.31151546176354794  DataLoggingVariableName=ScopeData3
  To Workspace1 : ToWorkspace  VariableName=pitch  SaveFormat=Timeseries  SampleTime=-1
      settings: Save2DSignal=2-D array (concatenate along first dimension)
  To Workspace2 : ToWorkspace  VariableName=roll  SaveFormat=Timeseries  SampleTime=-1
      settings: Save2DSignal=2-D array (concatenate along first dimension)
  To Workspace4 : ToWorkspace  VariableName=yaw  SaveFormat=Timeseries  SampleTime=-1
      settings: Save2DSignal=2-D array (concatenate along first dimension)
  Yaw_true : Scope
      settings: TimeSpan=600  ActiveDisplayYMinimum=-0.30825710918795335  ActiveDisplayYMaximum=0.31512173774753749  DataLoggingVariableName=ScopeData2
  Roll : Outport
  Pitch : Outport  Port=2
  "Yaw " : Outport  Port=3
  ORF2BODY : Outport  Port=4
  ORF2ECI : Outport  Port=5
  wires:
  MATLAB Function/3(yaw) -> "Yaw "/1, Gain1/1
  MATLAB Function/1(roll) -> Gain7/1, Roll/1
  "Attitude Quaternion "/1 -> R(IRF->BRF)/1(q)
  Measured ECI vel [km/s]/1 -> Mo/2(V (km/s) [ECI])
  Gain1/1 -> Yaw_true/1, To Workspace4/1  "Yaw"
  MATLAB Function/2(pitch) -> Pitch/1, Gain9/1
  Matrix Multiply/1 -> ORF2BODY/1, MATLAB Function/1(DCM)
  Gain7/1 -> To Workspace2/1, Roll_true/1  "Roll"
  Mo/1(Out1) -> ORF2ECI/1, Matrix Multiply/2
  Gain9/1 -> To Workspace1/1, Pitch_true/1  "Pitch"
  R(IRF->BRF)/1(R) -> Matrix Multiply/1
  Measured ECI pos [km]/1 -> Mo/1(X (km) [ECI]), Altitude Check/1(In1)

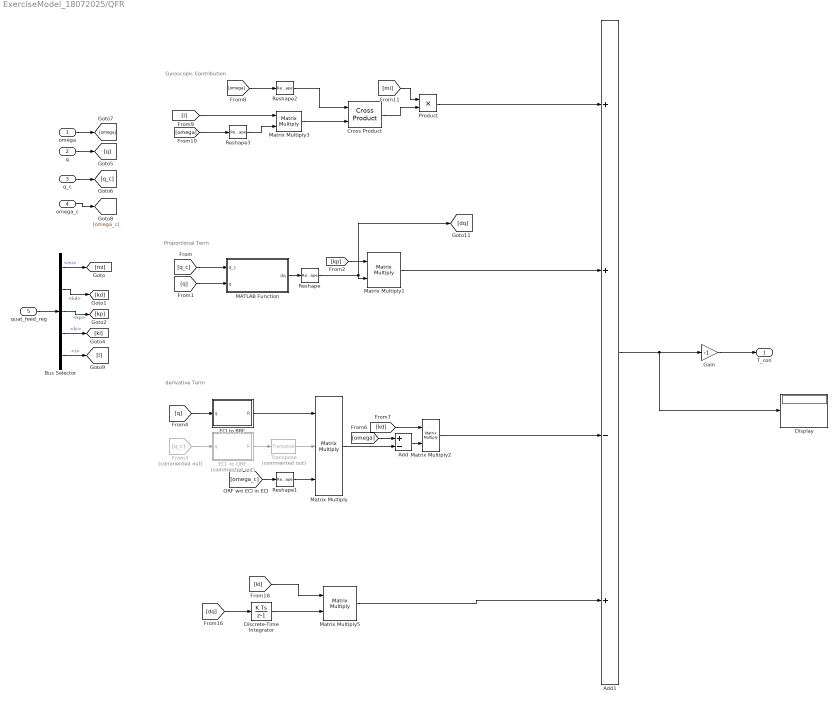
== system ExerciseModel_18072025/QFR ==
  note: Gyroscopic Contribution
  note: derivative Term
  note: Proportional Term
  omega : Inport
  q : Inport  Port=2
  q_c : Inport  Port=3
  omega_c : Inport  Port=4
  quat_feed_reg : Inport  Port=5
  Add : Sum  Inputs=+-
  Add1 : Sum  Inputs=++-+
  Bus Selector : BusSelector  OutputSignals=mi,kd,kp,ki,I
  Cross Product : matrix_library/Cross Product
  Discrete-Time Integrator : DiscreteIntegrator  InitialCondition=zeros(3,1)  ICPrevOutput=DiscIntNeverNeededParam  ICPrevScaledInput=DiscIntNeverNeededParam
  Display : Display
  ECI  to ORF : MATLAB Function  Commented=on  TreatAsAtomicUnit=on
  ECI to BRF : MATLAB Function  TreatAsAtomicUnit=on
  From3 : From  Commented=on  GotoTag=q_c
  Gain : Gain  Gain=-1
  MATLAB Function : MATLAB Function  TreatAsAtomicUnit=on
  Matrix Multiply : Product  Inputs=3  Multiplication=Matrix(*)
  Matrix Multiply{1..3,5} (4 alike) : Product  Multiplication=Matrix(*)
  Product : Product
  Reshape{,1..3} (4 alike) : Reshape  OutputDimensionality=Column vector (2-D)
  Transpose : matrix_library/Transpose  Commented=on
  T_con : Outport
  wires:
  quat_feed_reg/1 -> Bus Selector/1
  Bus Selector/1 -> [mi]  "<mi>"
  Bus Selector/2 -> [kd]  "<kd>"
  Bus Selector/3 -> [kp]  "<kp>"
  Bus Selector/4 -> [ki]  "<ki>"
  q/1 -> [q]
  q_c/1 -> [q_c]
  omega/1 -> [omega]
  omega_c/1 -> [omega_c]
  [q_c] -> MATLAB Function/1(q_c)
  [q] -> MATLAB Function/2(q)
  MATLAB Function/1(dq) -> Reshape/1
  From3/1 -> ECI  to ORF/1(q)
  ECI  to ORF/1(R) -> Transpose/1
  Transpose/1 -> Matrix Multiply/2
  [q] -> ECI to BRF/1(q)
  ECI to BRF/1(R) -> Matrix Multiply/1
  [omega_c] -> Reshape1/1
  Reshape1/1 -> Matrix Multiply/3
  Matrix Multiply/1 -> Add/2
  [omega] -> Add/1
  [kp] -> Matrix Multiply1/1
  Reshape/1 -> [dq], Matrix Multiply1/2
  Add/1 -> Matrix Multiply2/2
  [kd] -> Matrix Multiply2/1
  Bus Selector/5 -> [I]  "<I>"
  [omega] -> Reshape2/1
  Reshape2/1 -> Cross Product/1
  [omega] -> Reshape3/1
  [I] -> Matrix Multiply3/1
  Reshape3/1 -> Matrix Multiply3/2
  Matrix Multiply3/1 -> Cross Product/2
  Cross Product/1 -> Product/2
  [mi] -> Product/1
  Product/1 -> Add1/1
  Matrix Multiply1/1 -> Add1/2
  Matrix Multiply2/1 -> Add1/3
  Add1/1 -> Display/1, Gain/1
  [dq] -> Discrete-Time Integrator/1
  Discrete-Time Integrator/1 -> Matrix Multiply5/2
  [ki] -> Matrix Multiply5/1
  Matrix Multiply5/1 -> Add1/4
  Gain/1 -> T_con/1

== system ExerciseModel_18072025/S direction, B components in BRF and ECI ==
  R_ECIBRF : Inport
  Sdir_ECI_vec : Inport  Port=2
  B_ECI_vec : Inport  Port=3
  eclipse_flag : Inport  Port=4
  Constant : Constant  Value=Magnetometers_number
  Constant1 : Constant  Value=Sun_sensors
  Constant2 : Constant  Value=FOV
  MATLAB Function : MATLAB Function  TreatAsAtomicUnit=on  SystemSampleTime=step_size
  MATLAB Function1 : MATLAB Function  TreatAsAtomicUnit=on  SystemSampleTime=step_size
  Sdir_ECI_matrix : Outport
  Sdir_BRF_matrix : Outport  Port=2
  Bdir_ECI_matrix : Outport  Port=3
  B_BRF_matrix : Outport  Port=4
  wires:
  Sdir_ECI_vec/1 -> MATLAB Function/1(Sdir_ECI_vec)
  R_ECIBRF/1 -> MATLAB Function1/1(R_ECIBRF), MATLAB Function/2(R_ECIBRF)
  B_ECI_vec/1 -> MATLAB Function1/2(B_ECI_vec)
  MATLAB Function/1(Sdir_ECI_matrix) -> Sdir_ECI_matrix/1
  MATLAB Function/2(Sdir_BRF_matrix) -> Sdir_BRF_matrix/1
  MATLAB Function1/1(Bdir_ECI_matrix) -> Bdir_ECI_matrix/1
  MATLAB Function1/2(B_BRF_matrix) -> B_BRF_matrix/1
  Constant/1 -> MATLAB Function1/3(Magnetometers_number)
  Constant1/1 -> MATLAB Function/3(Sun_sensors)
  Constant2/1 -> MATLAB Function/4(FOV)
  eclipse_flag/1 -> MATLAB Function/5(eclipse_flag)

== system ExerciseModel_18072025/Sensors ==
  Sdir_BRF_matrix : Inport
  B_BRF_matrix : Inport  Port=2
  omega_ECI : Inport  Port=3
  Angular velocity noise : MATLAB Function  TreatAsAtomicUnit=on  SystemSampleTime=step_size
  Constant : Constant  Value=MeanangularSun
  Constant1 : Constant  Value=SigmaangularSun
  Constant2 : Constant  Value=Sigma_cart_Mag
  Constant3 : Constant  Value=Mean_cart_Mag
  Constant4 : Constant  Value=Bias
  Constant5 : Constant  Value=ARW
  Constant6 : Constant  Value=step_size
  Magnetic field noise : MATLAB Function  TreatAsAtomicUnit=on  SystemSampleTime=step_size
  Sun direction noise : MATLAB Function  TreatAsAtomicUnit=on  SystemSampleTime=step_size
  Sdir_BRF_matrix_noise : Outport
  Bdir_BRF_matrix_noise : Outport  Port=2
  B_BRF_matrix_noise : Outport  Port=3
  omega_noise : Outport  Port=4
  wires:
  Sdir_BRF_matrix/1 -> Sun direction noise/1(Sdir_BRF_matrix)
  B_BRF_matrix/1 -> Magnetic field noise/1(B_BRF_matrix)
  Sun direction noise/1(Sdir_BRF_matrix_noise) -> Sdir_BRF_matrix_noise/1
  Constant/1 -> Sun direction noise/2(MeanangularSun)
  Constant1/1 -> Sun direction noise/3(SigmaangularSun)
  Constant2/1 -> Magnetic field noise/3(Sigma_cart_Mag)
  Constant3/1 -> Magnetic field noise/2(Mean_cart_Mag)
  Magnetic field noise/1(B_BRF_matrix_noise) -> B_BRF_matrix_noise/1
  Magnetic field noise/2(Bdir_BRF_matrix_noise) -> Bdir_BRF_matrix_noise/1
  Constant4/1 -> Angular velocity noise/2(Bias_omega)
  Constant5/1 -> Angular velocity noise/3(ARW)
  Constant6/1 -> Angular velocity noise/4(dt)
  omega_ECI/1 -> Angular velocity noise/1(omega_true)
  Angular velocity noise/1(omega_noise) -> omega_noise/1

== system ExerciseModel_18072025/Spacecraft Dynamics Model ==
  f : Inport
  drag : Inport  Port=2
  h_w : Inport  Port=3
  T_control : Inport  Port=4
  T_ext : Inport  Port=5
  Constant : Constant  Value=Sat_mass
  Constant1 : Constant  Value=Sat_Inertia
  Equations of motion of the spacecraft : MATLAB Function  TreatAsAtomicUnit=on
  dfdt : Outport
  wires:
  T_ext/1 -> Equations of motion of the spacecraft/7(T_ext)
  T_control/1 -> Equations of motion of the spacecraft/6(T_control)
  h_w/1 -> Equations of motion of the spacecraft/5(h_w)
  drag/1 -> Equations of motion of the spacecraft/2(drag)
  f/1 -> Equations of motion of the spacecraft/1(f)
  Equations of motion of the spacecraft/1(dfdt) -> dfdt/1
  Constant/1 -> Equations of motion of the spacecraft/3(m)
  Constant1/1 -> Equations of motion of the spacecraft/4(I)

== system ExerciseModel_18072025/Sun_B angle ==
  Sdir_ECI_vec : Inport
  B_ECI_vec : Inport  Port=2
  Action Port : ActionPort  ActionPortLabel=if(u1 == 1)
  Acos : Trigonometry  Operator=acos
  Divide : Product  Inputs=*/
  Dot Product : DotProduct  OutDataTypeStr=Inherit: Inherit via internal rule
  Dot Product1 : DotProduct  OutDataTypeStr=Inherit: Inherit via internal rule
  Gain : Gain  Gain=180/pi
  Sqrt : Sqrt
  angle_SB : Outport
  wires:
  Acos/1 -> Gain/1
  Dot Product/1 -> Acos/1
  Dot Product1/1 -> Sqrt/1
  Sqrt/1 -> Divide/2
  B_ECI_vec/1 -> Divide/1, Dot Product1/1, Dot Product1/2
  Divide/1 -> Dot Product/2
  Sdir_ECI_vec/1 -> Dot Product/1
  Gain/1 -> angle_SB/1

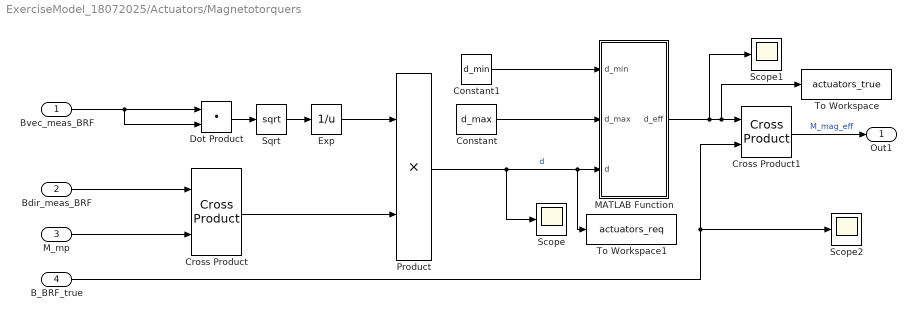
== system ExerciseModel_18072025/Actuators/Magnetotorquers ==
  Bvec_meas_BRF : Inport
  Bdir_meas_BRF : Inport  Port=2
  M_mp : Inport  Port=3
  B_BRF_true : Inport  Port=4
  Constant : Constant  Value=d_max
  Constant1 : Constant  Value=d_min
  Cross Product : matrix_library/Cross Product
  Cross Product1 : matrix_library/Cross Product
  Dot Product : DotProduct  OutDataTypeStr=Inherit: Inherit via internal rule
  Exp : Math  Operator=reciprocal
  MATLAB Function : MATLAB Function  TreatAsAtomicUnit=on
  Product : Product
  Scope : Scope
      settings: ActiveDisplayYMinimum=-0.652674795620126  ActiveDisplayYMaximum=0.63384775110992186  DataLoggingVariableName=ScopeData20
  Scope1 : Scope
      settings: ActiveDisplayYMinimum=-0.3625  ActiveDisplayYMaximum=0.3625  DataLoggingVariableName=ScopeData21
  Scope2 : Scope
      settings: ActiveDisplayYMinimum=-7.7586179310404373E-5  ActiveDisplayYMaximum=3.13681877624174E-5  DataLoggingVariableName=ScopeData36
  Sqrt : Sqrt
  To Workspace : ToWorkspace  VariableName=actuators_true  SaveFormat=Timeseries  SampleTime=-1
  To Workspace1 : ToWorkspace  VariableName=actuators_req  SaveFormat=Timeseries  SampleTime=-1
  Out1 : Outport
  wires:
  M_mp/1 -> Cross Product/2
  Bvec_meas_BRF/1 -> Dot Product/2, Dot Product/1
  Dot Product/1 -> Sqrt/1
  Sqrt/1 -> Exp/1
  Bdir_meas_BRF/1 -> Cross Product/1
  Cross Product/1 -> Product/2
  Exp/1 -> Product/1
  Product/1 -> Scope/1, To Workspace1/1, MATLAB Function/3(d)  "d"
  Constant/1 -> MATLAB Function/2(d_max)
  Constant1/1 -> MATLAB Function/1(d_min)
  MATLAB Function/1(d_eff) -> Scope1/1, To Workspace/1, Cross Product1/1
  Cross Product1/1 -> Out1/1  "M_mag_eff"
  B_BRF_true/1 -> Scope2/1, Cross Product1/2

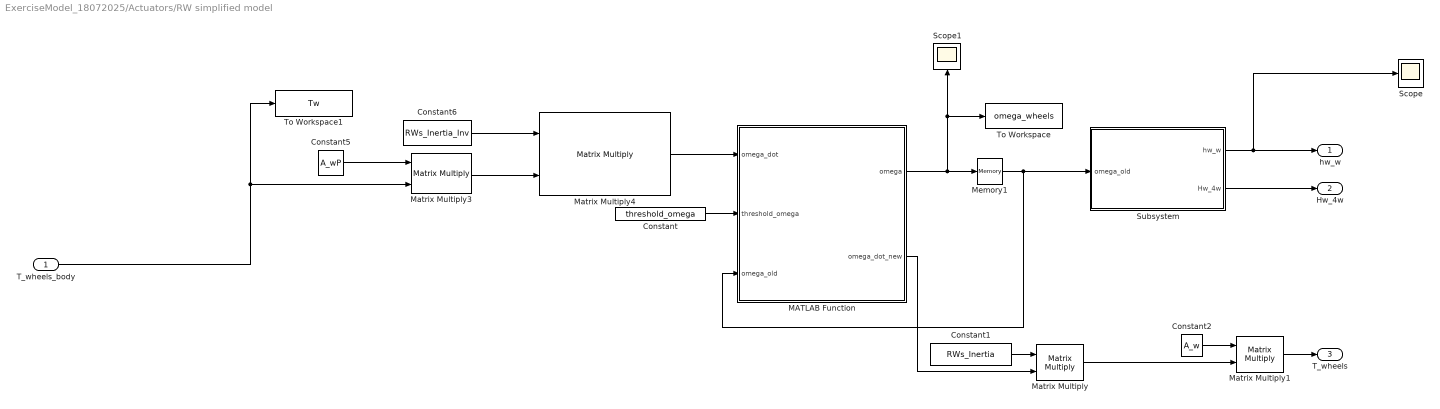
== system ExerciseModel_18072025/Actuators/RW simplified model ==
  T_wheels_body : Inport
  Constant : Constant  Value=threshold_omega
  Constant1 : Constant  Value=RWs_Inertia
  Constant2 : Constant  Value=A_w
  Constant5 : Constant  Value=A_wP
  Constant6 : Constant  Value=RWs_Inertia_Inv
  MATLAB Function : MATLAB Function  TreatAsAtomicUnit=on
  Matrix Multiply{,1,3..4} (4 alike) : Product  Multiplication=Matrix(*)
  Memory1 : Memory  InitialCondition=zeros(4,1)
  Scope : Scope
      settings: DataLoggingVariableName=ScopeData2
  Scope1 : Scope
      settings: ActiveDisplayYMinimum=-1047.197551  ActiveDisplayYMaximum=1047.197551  DataLoggingVariableName=ScopeData22
  Subsystem : Subsystem
  To Workspace : ToWorkspace  VariableName=omega_wheels  SaveFormat=Timeseries  SampleTime=-1
  To Workspace1 : ToWorkspace  VariableName=Tw  SaveFormat=Structure With Time  SampleTime=-1
  hw_w : Outport
  Hw_4w : Outport  Port=2
  T_wheels : Outport  Port=3
  wires:
  Constant5/1 -> Matrix Multiply3/1
  T_wheels_body/1 -> To Workspace1/1, Matrix Multiply3/2
  Constant6/1 -> Matrix Multiply4/1
  Matrix Multiply3/1 -> Matrix Multiply4/2
  Matrix Multiply4/1 -> MATLAB Function/1(omega_dot)
  Memory1/1 -> MATLAB Function/3(omega_old), Subsystem/1(omega_old)
  MATLAB Function/1(omega) -> Memory1/1, To Workspace/1, Scope1/1
  Subsystem/2(Hw_4w) -> Hw_4w/1
  Subsystem/1(hw_w) -> hw_w/1, Scope/1
  MATLAB Function/2(omega_dot_new) -> Matrix Multiply/2
  Constant1/1 -> Matrix Multiply/1
  Matrix Multiply/1 -> Matrix Multiply1/2
  Constant2/1 -> Matrix Multiply1/1
  Matrix Multiply1/1 -> T_wheels/1
  Constant/1 -> MATLAB Function/2(threshold_omega)

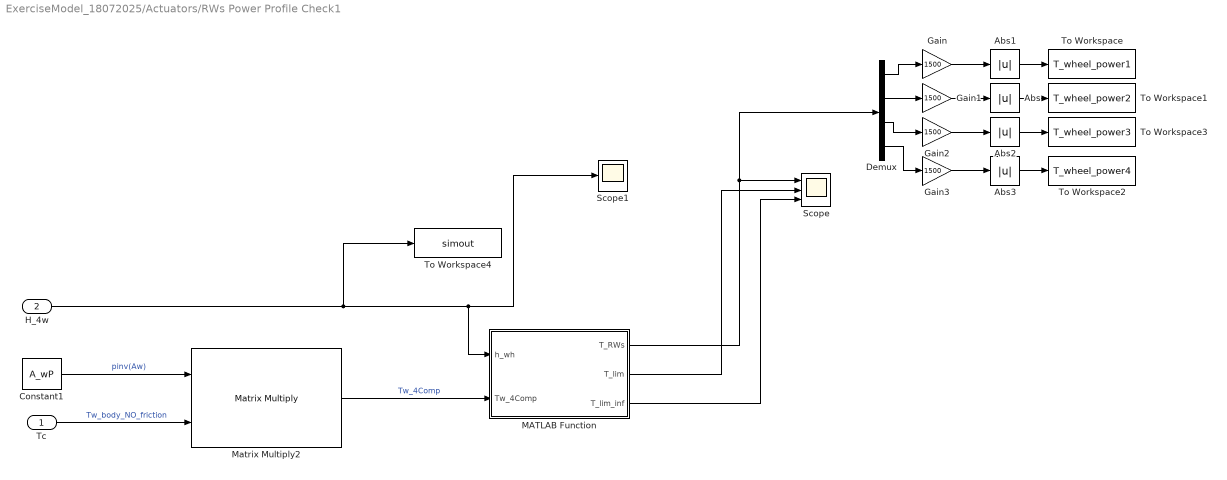
== system ExerciseModel_18072025/Actuators/RWs Power Profile Check1 ==
  Tc : Inport
  H_4w : Inport  Port=2
  Abs{,1..3} (4 alike) : Abs  SaturateOnIntegerOverflow=off
  Constant1 : Constant  Value=A_wP
  Demux : Demux
  Gain{,1..3} (4 alike) : Gain  Gain=1500
  MATLAB Function : MATLAB Function  TreatAsAtomicUnit=on
  Matrix Multiply2 : Product  Multiplication=Matrix(*)
  Scope : Scope  NumInputPorts=3
      settings: ActiveDisplayYMinimum=-0.0067  ActiveDisplayYMaximum=0.00648
  Scope1 : Scope
      settings: ActiveDisplayYMinimum=-0.12077  ActiveDisplayYMaximum=0.09415  DataLoggingVariableName=ScopeData2
  To Workspace : ToWorkspace  VariableName=T_wheel_power1  SaveFormat=Timeseries  SampleTime=-1
  To Workspace1 : ToWorkspace  VariableName=T_wheel_power2  SaveFormat=Timeseries  SampleTime=-1
  To Workspace2 : ToWorkspace  VariableName=T_wheel_power4  SaveFormat=Timeseries  SampleTime=-1
  To Workspace3 : ToWorkspace  VariableName=T_wheel_power3  SaveFormat=Timeseries  SampleTime=-1
  To Workspace4 : ToWorkspace  VariableName=simout  SaveFormat=Timeseries  SampleTime=-1
  wires:
  Constant1/1 -> Matrix Multiply2/1  "pinv(Aw)"
  Matrix Multiply2/1 -> MATLAB Function/2(Tw_4Comp)  "Tw_4Comp"
  Tc/1 -> Matrix Multiply2/2  "Tw_body_NO_friction"
  MATLAB Function/1(T_RWs) -> Demux/1, Scope/1
  H_4w/1 -> To Workspace4/1, Scope1/1, MATLAB Function/1(h_wh)
  MATLAB Function/3(T_lim_inf) -> Scope/3
  Demux/2 -> Gain1/1
  Demux/1 -> Gain/1
  Demux/3 -> Gain2/1
  Demux/4 -> Gain3/1
  Gain2/1 -> Abs2/1
  Gain1/1 -> Abs/1
  Gain/1 -> Abs1/1
  Gain3/1 -> Abs3/1
  MATLAB Function/2(T_lim) -> Scope/2
  Abs1/1 -> To Workspace/1
  Abs/1 -> To Workspace1/1
  Abs3/1 -> To Workspace2/1
  Abs2/1 -> To Workspace3/1

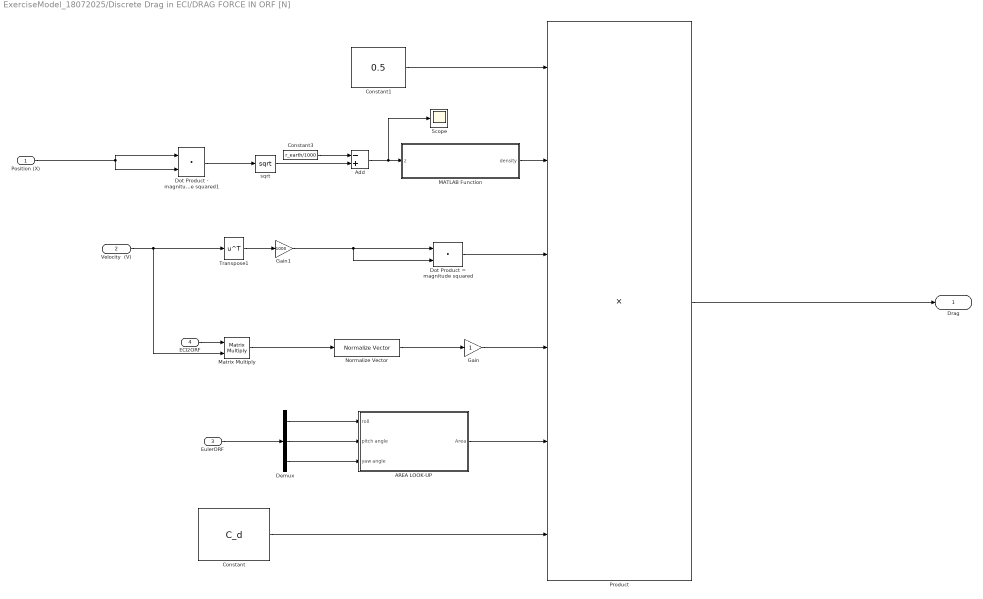
== system ExerciseModel_18072025/Discrete Drag in ECI/DRAG FORCE IN ORF [N] ==
  Position (X) : Inport
  Velocity  (V) : Inport  Port=2
  EulerORF : Inport  Port=3
  ECI2ORF : Inport  Port=4
  AREA LOOK-UP : Subsystem
  Add : Sum  Inputs=-+
  Constant : Constant  Value=C_d
  Constant1 : Constant  Value=0.5
  Constant3 : Constant  Value=r_earth/1000
  Demux : Demux  Outputs=3
  Dot Product - magnitude squared1 : DotProduct  OutDataTypeStr=Inherit: Inherit via internal rule
  Dot Product = magnitude squared : DotProduct  OutDataTypeStr=Inherit: Inherit via internal rule
  Gain : Gain
  Gain1 : Gain  Gain=1000
  MATLAB Function : MATLAB Function  TreatAsAtomicUnit=on
  Matrix Multiply : Product  Multiplication=Matrix(*)
  Normalize Vector : vrlib/Utilities/Normalize Vector  maxzero=0
  Product : Product  Inputs=6
  Scope : Scope
      settings: ActiveDisplayYMinimum=296.75857  ActiveDisplayYMaximum=313.34132
  Transpose1 : Math  Operator=transpose  SignedPower=on
  sqrt : Math  Operator=sqrt  SignedPower=on
  Drag : Outport
  wires:
  sqrt/1 -> Add/2
  Add/1 -> Scope/1, MATLAB Function/1(z)
  MATLAB Function/1(density) -> Product/2
  Constant3/1 -> Add/1
  Demux/3 -> AREA LOOK-UP/3(yaw angle)
  Demux/2 -> AREA LOOK-UP/2(pitch angle)
  Demux/1 -> AREA LOOK-UP/1(roll)
  Product/1 -> Drag/1
  Dot Product = magnitude squared/1 -> Product/3
  Gain/1 -> Product/4
  Normalize Vector/1 -> Gain/1
  Constant1/1 -> Product/1
  AREA LOOK-UP/1(Area) -> Product/5
  Constant/1 -> Product/6
  Velocity  (V)/1 -> Matrix Multiply/2, Transpose1/1
  Transpose1/1 -> Gain1/1
  Position (X)/1 -> Dot Product - magnitude squared1/1, Dot Product - magnitude squared1/2
  Dot Product - magnitude squared1/1 -> sqrt/1
  EulerORF/1 -> Demux/1
  ECI2ORF/1 -> Matrix Multiply/1
  Matrix Multiply/1 -> Normalize Vector/1
  Gain1/1 -> Dot Product = magnitude squared/1, Dot Product = magnitude squared/2

== system ExerciseModel_18072025/External Disturbance Torques/AeroTorque in BRF ==
  note: Velocity squared
  POS ECI [km] : Inport
  VEL ECI [km] : Inport  Port=2
  R(ORF->BRF) : Inport  Port=3
  ORF_Eul : Inport  Port=4
  Add : Sum  Inputs=-+
  Constant2 : Constant  Value=r_earth
  Conversion : Gain  Gain=1000
  Demux : Demux  Outputs=3
  Dot Prod. : DotProduct  OutDataTypeStr=Inherit: Inherit via internal rule
  Dot Product = magnitude squared : DotProduct  OutDataTypeStr=Inherit: Inherit via internal rule
  Gain : Gain  Gain=1/1000
  MATLAB Function : MATLAB Function  TreatAsAtomicUnit=on
  Product2 : Product  RndMeth=Zero
  Product3 : Product  RndMeth=Zero
  TORQUE FACTOR : Subsystem
  Transpose1 : Math  Operator=transpose  SignedPower=on
  product 3 : Product  Multiplication=Matrix(*)  RndMeth=Zero
  sqrt : Math  Operator=sqrt  SignedPower=on
  Aero. Torque (N.m) : Outport
  wires:
  sqrt/1 -> Add/2
  Add/1 -> MATLAB Function/1(z)
  Constant2/1 -> Gain/1
  Demux/3 -> TORQUE FACTOR/3(yaw angle)
  Demux/2 -> TORQUE FACTOR/2(pitch angle)
  Demux/1 -> TORQUE FACTOR/1(roll)
  Product2/1 -> Aero. Torque (N.m)/1
  Dot Product = magnitude squared/1 -> Product3/2
  MATLAB Function/1(density) -> Product3/1
  VEL ECI [km]/1 -> Conversion/1
  Transpose1/1 -> Dot Product = magnitude squared/1, Dot Product = magnitude squared/2
  TORQUE FACTOR/1(T_comp) -> product 3/2  "torque_factor_components_ORF"
  product 3/1 -> Product2/1
  Product3/1 -> Product2/2
  Dot Prod./1 -> sqrt/1
  POS ECI [km]/1 -> Dot Prod./2, Dot Prod./1
  R(ORF->BRF)/1 -> product 3/1
  ORF_Eul/1 -> Demux/1
  Conversion/1 -> Transpose1/1
  Gain/1 -> Add/1

== system ExerciseModel_18072025/External Disturbance Torques/Gravity Gradient Model ==
  Pos ECI [km] : Inport
  R(IRF->BRF) : Inport  Port=2
  Constant : Constant  Value=3*m_earth*G_earth
  Constant1 : Constant  Value=Sat_Inertia
  Cross Product : matrix_library/Cross Product
  Divide : Product  Inputs=*/
  Dot Product : DotProduct  OutDataTypeStr=Inherit: Inherit via internal rule
  Gain : Gain  Gain=-1
  Gain1 : Gain  Gain=-1
  Gain2 : Gain  Gain=1000
  Math Function : Math  Operator=square  SignedPower=on
  Product : Product  Multiplication=Matrix(*)  RndMeth=Zero
  Prouct : Product  RndMeth=Zero
  Vector Normal : vrlib/Utilities/Normalize Vector  maxzero=0
  "product " : Product  Multiplication=Matrix(*)  RndMeth=Zero
  Gravity Gradient (N.m) : Outport
  wires:
  Divide/1 -> Prouct/2
  Constant/1 -> Divide/1
  Math Function/1 -> Divide/2
  Vector Normal/1 -> Gain/1
  Cross Product/1 -> Gravity Gradient (N.m)/1
  Dot Product/1 -> Math Function/1
  Product/1 -> Cross Product/2
  Constant1/1 -> Product/1
  "product "/1 -> Vector Normal/1, Gain1/1
  Gain1/1 -> Prouct/1
  Pos ECI [km]/1 -> Gain2/1
  Gain/1 -> Product/2
  Prouct/1 -> Cross Product/1
  R(IRF->BRF)/1 -> "product "/1
  Gain2/1 -> "product "/2, Dot Product/1, Dot Product/2
